simulink model "Lab05_Bai02"  (R2019a)
settings: Solver=VariableStepAuto  StartTime=0.0  StopTime=0.05  RelTol=1e-3
libraries: commanapbnd3 x4
settings Model: Creator=nth22  LastModifiedBy=nth22

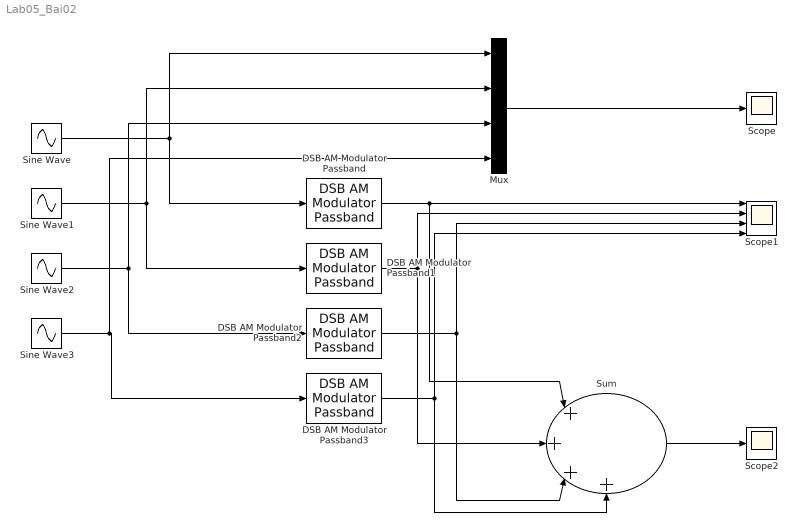
== system Lab05_Bai02 ==
  DSB AM Modulator Passband{,1..3} (4 alike) : commanapbnd3/DSB AM Modulator Passband  Fc=300  Ph=0  Offset=1
      settings: SourceProductName=Communications Toolbox  SourceProductBaseCode=CM
  Mux : Mux
  Scope : Scope
  Scope1 : Scope  NumInputPorts=4
  Scope2 : Scope
  Sine Wave : Sin  Frequency=100*pi  SampleTime=0.0001
  Sine Wave1 : Sin  Frequency=100*pi  Phase=pi/4  SampleTime=0.0001
  Sine Wave2 : Sin  Frequency=100*pi  Phase=pi/2  SampleTime=0.0001
  Sine Wave3 : Sin  Frequency=100*pi  Phase=0.75*pi  SampleTime=0.0001
  Sum : Sum  Inputs=|++++
  wires:
  Sine Wave/1 -> Mux/1, DSB AM Modulator Passband/1
  Sine Wave1/1 -> DSB AM Modulator Passband1/1, Mux/2
  Sine Wave2/1 -> Mux/3, DSB AM Modulator Passband2/1
  Sine Wave3/1 -> Mux/4, DSB AM Modulator Passband3/1
  Mux/1 -> Scope/1
  DSB AM Modulator Passband/1 -> Sum/1, Scope1/1
  DSB AM Modulator Passband1/1 -> Sum/2, Scope1/2
  DSB AM Modulator Passband2/1 -> Sum/3, Scope1/3
  DSB AM Modulator Passband3/1 -> Scope1/4, Sum/4
  Sum/1 -> Scope2/1
